simulink model "sldemo_suspn_3dof"  (R2018a)
settings: Solver=ode45  StartTime=0.0  StopTime=100  MaxStep=0.001  RelTol=1e-3  AbsTol=1e-6
PreLoadFcn:
  | sldemo_suspn_3dof_data
undefined symbols (not defined in the file or in its folder): Cr, g, Ixx, Iyy, Kf, Kr, L, Mb, sigbuilder_block, W
Description:
  | Automotive Suspension
  | 
  | This demo describes a simplified car suspension model in three degrees of
  | freedom (DoF): pitch, yaw and vertical displacement. The demo provides a description of the model to
  | show how simulation can be used for investigating ride characteristics. The Signal Builder block was used to
  | capture different road profiles to test the suspension against.
settings Model: FPTRunName=Active  ModifiedByFormat=The MathWorks Inc.  ExtModeTrigMode=oneshot  ExtModeArmWhenConnect=off  ExtModeAutoUpdateStatusClock=off  TunableVars=Cf,Mb  TunableVarsStorageClass=Auto,Auto  TunableVarsTypeQualifier=,  Creator=The MathWorks, Inc.  LastModifiedBy=The MathWorks Inc.
settings SolverCC: AutoScaleAbsTol=off
settings DataIOCC: InitialState=x0  SaveFormat=Array  SaveOutput=off  DSMLogging=off  SaveTime=off  ReturnWorkspaceOutputs=on  StateSaveName=x  ReturnWorkspaceOutputsName=simout
settings OptimizationCC: BooleanDataType=off  DefaultParameterBehavior=Inlined  InlineInvariantSignals=on  ExpressionDepthLimit=2147483647  InitFltsAndDblsToZero=on  LifeSpan=inf  BufferReusableBoundary=off
settings DebuggingCC: SaveWithParameterizedLinksMsg=none  SignalResolutionControl=TryResolveAllWithWarning  MultiTaskDSMMsg=warning  SigSpecEnsureSampleTimeMsg=none  IntegerOverflowMsg=none  FcnCallInpInsideContextMsg=warning  BusObjectLabelMismatch=none  StateNameClashWarn=warning  SFUnexpectedBacktrackingDiag=warning  SFNoUnconditionalDefaultTransitionDiag=warning  SFExecutionAtInitializationDiag=none  IntegerSaturationMsg=none
settings HardwareCC: ProdBitPerPointer=32  ProdBitPerSizeT=32  ProdBitPerPtrDiffT=32  ProdLargestAtomicFloat=None  ProdIntDivRoundTo=Undefined  ProdEndianess=Unspecified  ProdWordSize=32  ProdHWDeviceType=32-bit Generic
settings ModelReferenceCC: PropagateSignalLabelsOutOfModel=off
settings RTWCC: Description=Generic Real-Time Target
settings CodeAppCC: StateflowObjectComments=on
settings GRTTargetCC: TargetFcnLib=ansi_tfl_tmw.mat  TargetLangStandard=C89/C90 (ANSI)  GeneratePreprocessorConditionals=Disable all  CombineOutputUpdateFcns=off  GRTInterface=on
settings ConfigComp: CovMetricSettings=dw  CovHtmlReporting=on  CovSaveCumulativeToWorkspaceVar=on  CovSaveSingleToWorkspaceVar=on  CovExternalEMLEnable=off  CovSFcnEnable=off

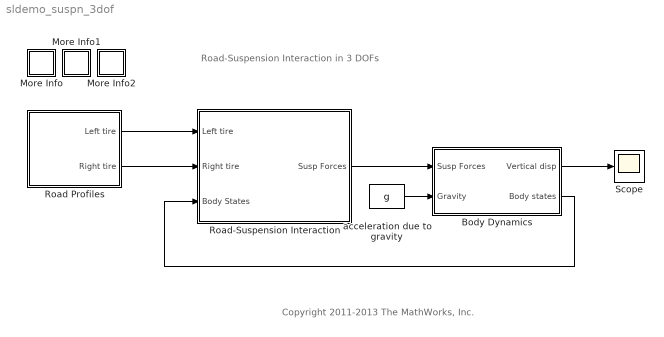
== system sldemo_suspn_3dof ==
  note: Road-Suspension Interaction in 3 DOFs
  note: Copyright 2011-2013 The MathWorks, Inc.
  Body Dynamics : Subsystem
  More Info : Subsystem
      settings: OpenFcn=helpview(fullfile(docroot,'simulink','helptargets.map'),'sldemo_parsim_testcase_suspn');
      mask Display: disp('?')
  More Info1 : Subsystem
      settings: OpenFcn=helpview(fullfile(docroot,'simulink','helptargets.map'),'sldemo_parsim_paramsweep_suspn');
      mask Display: disp('?')
  More Info2 : Subsystem
      settings: OpenFcn=helpview(fullfile(docroot,'simulink','helptargets.map'),'sldemo_parsim_paramsweep_suspn_raccel');
      mask Display: disp('?')
  Road Profiles : Subsystem  Tag=STV Subsys  LoadFcn=sigbuilder_block('load');  StartFcn=sigbuilder_block('start');  StopFcn=sigbuilder_block('stop');  ClipboardFcn=sigbuilder_block('clipboard');  mask(Sigbuilder block){tuvar=[0:10]}
      mask help: Create and generate interchangeable groups of signals whose waveforms are piecewise linear.
      mask init:
      | if ~strcmp(get_param(bdroot(gcbh),'SimulationStatus'),'stopped') tuvar = sigbuilder_block('maskInit'); end
      settings: CopyFcn=sigbuilder_block('copy');  DeleteFcn=sigbuilder_block('delete');  ModelCloseFcn=sigbuilder_block('modelClose');  PreSaveFcn=sigbuilder_block('preSave');  PauseFcn=sigbuilder_block('pause')  ContinueFcn=sigbuilder_block('continue')  NameChangeFcn=sigbuilder_block('namechange');  OpenFcn=sigbuilder_block('open',[108.621 149.586 549.931 399.724 ]);  CloseFcn=sigbuilder_block('close');
      mask Display: plot(0, 0, 100, 100,[2, 2, 32, 32, 2], [68, 8, 8, 68, 68],[32, 2], [38, 38], [32, 19, 2],[53, 60, 44], [32, 17, 17, 2],[16, 16, 31, 31]);txt = getActiveGroup(gcbh);text(2, 100, txt,'verticalAlignment', 'top');
  Road-Suspension Interaction : Subsystem  mask{Kf=Kf, Cf=150, Kr=Kr, Cr=Cr}
      mask prompts: Kf "Front susp. stiffness"; Cf "Front susp. damping"; Kr "Rear susp. stiffness"; Cr "Rear susp. damping"
  Scope : Scope
  acceleration due to gravity : Constant  Value=g
  wires:
  Road-Suspension Interaction/1(Susp Forces) -> Body Dynamics/1(Susp Forces)
  Road Profiles/1(Left tire) -> Road-Suspension Interaction/1("Left tire ")
  Road Profiles/2(Right tire) -> Road-Suspension Interaction/2(Right tire)
  Body Dynamics/2(Body states) -> Road-Suspension Interaction/3(Body States)
  Body Dynamics/1(Vertical disp) -> Scope/1
  acceleration due to gravity/1 -> Body Dynamics/2(Gravity)

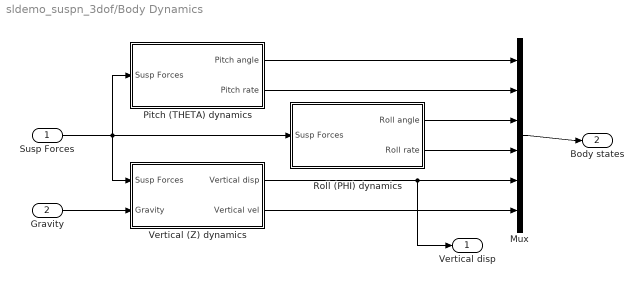
== system sldemo_suspn_3dof/Body Dynamics ==
  Susp Forces : Inport
  Gravity : Inport  Port=2
  Mux : Mux  Inputs=6
  Pitch (THETA) dynamics : Subsystem
  Roll (PHI) dynamics : Subsystem
  Vertical (Z) dynamics : Subsystem
  Vertical disp : Outport
  Body states : Outport  Port=2
  wires:
  Mux/1 -> Body states/1
  Pitch (THETA) dynamics/1(Pitch angle) -> Mux/1
  Pitch (THETA) dynamics/2(Pitch rate) -> Mux/2
  Roll (PHI) dynamics/1(Roll angle) -> Mux/3
  Roll (PHI) dynamics/2(Roll rate) -> Mux/4
  Vertical (Z) dynamics/1(Vertical disp) -> Mux/5, Vertical disp/1
  Vertical (Z) dynamics/2(Vertical vel) -> Mux/6
  Susp Forces/1 -> Pitch (THETA) dynamics/1(Susp Forces), Roll (PHI) dynamics/1(Susp Forces), Vertical (Z) dynamics/1(Susp Forces)
  Gravity/1 -> Vertical (Z) dynamics/2(Gravity)

== system sldemo_suspn_3dof/More Info ==

== system sldemo_suspn_3dof/More Info1 ==

== system sldemo_suspn_3dof/More Info2 ==

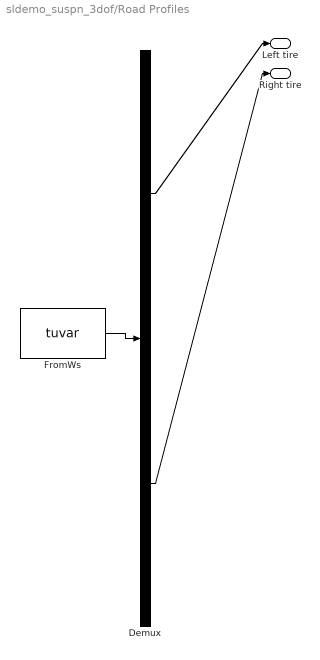
== system sldemo_suspn_3dof/Road Profiles ==
  Demux : Demux  Tag=STV Demux  Outputs=2
  FromWs : FromWorkspace  Tag=STV FromWs  VariableName=tuvar  SampleTime=0  OutputAfterFinalValue=Setting to zero
      SigBuilderData=|
      | common.afterFinalStr = 'Set to zero'
      | common.sampleTime = '0'
      | dataSet(1).timeRange = [0 102.3]
      | dataSet(1).name = 'Road1'
      | dataSet(2).timeRange = [0 102.3]
      | dataSet(2).name = 'Road2'
      | dataSet(3).timeRange = [0 102.3]
      | dataSet(3).name = 'Road3'
      | dataSet(4).timeRange = [0 102.3]
      | dataSet(4).name = 'Road4'
      | dataSet(5).timeRange = [0 102.3]
      | dataSet(5).name = 'Road5'
      | dataSet(6).timeRange = [0 102.3]
      | dataSet(6).name = 'Road6'
      | dataSet(7).timeRange = [0 102.3]
      | dataSet(7).name = 'Road7'
      | dataSet(8).timeRange = [0 102.3]
      | dataSet(8).name = 'Road8'
      | dataSet(9).timeRange = [0 102.3]
      | dataSet(9).name = 'Road9'
      | dataSet(10).timeRange = [0 102.3]
      | dataSet(10).name = 'Road10'
      | dataSet(11).timeRange = [0 102.3]
      | dataSet(11).name = 'Road11'
      | dataSet(12).timeRange = [0 102.3]
      | dataSet(12).name = 'Road12'
      | dataSet(13).timeRange = [0 102.3]
      | dataSet(13).name = 'Road13'
      | dataSet(14).timeRange = [0 102.3]
      | dataSet(14).name = 'Road14'
      | dataSet(15).timeRange = [0 102.3]
      | dataSet(15).name = 'Road15'
      | dataSet(16).timeRange = [0 102.3]
      | dataSet(16).name = 'Road16'
      | dataSet(17).timeRange = [0 102.3]
      | dataSet(17).name = 'Road17'
      | dataSet(18).timeRange = [0 102.3]
      | dataSet(18).name = 'Road18'
      | dataSet(19).timeRange = [0 102.3]
      | dataSet(19).name = 'Road19'
      | dataSet(20).timeRange = [0 102.3]
      | dataSet(20).name = 'Road20'
      | sbobj.Name = 'Signal Builder'
      | sbobj.Groups(1).Name = 'Road1'
      | sbobj.Groups(1).Signals(1).Name = 'Left tire'
      | sbobj.Groups(1).Signals(1).XData = [0 0.1 0.2 0.3 0.4 0.5 0.6 0.7 0.8 0.9 1 1.1 ... (1024 elements, 1x1024)]
      | sbobj.Groups(1).Signals(1).YData = [0.00473211644634 0.00467440555502 0.00464410099502 0.00454324182484 0.00445514799148 0.0043326490208 0.00423785066412 0.0042993177206 0.00422544735533 0.00410809626891 0.00412946729868 0.00411767616593 ... (1024 elements, 1x1024)]
      | sbobj.Groups(1).Signals(2).Name = 'Right tire'
      | sbobj.Groups(1).Signals(2).XData = [0 0.1 0.2 0.3 0.4 0.5 0.6 0.7 0.8 0.9 1 1.1 ... (1024 elements, 1x1024)]
      | sbobj.Groups(1).Signals(2).YData = [0.00528049577434 0.00509711727989 0.00506446595634 0.00501214877729 0.00490088724648 0.0049331354282 0.00486498626463 0.00475766732988 0.0047835078559 0.00468735204086 0.00453387383384 0.00439901634932 ... (1024 elements, 1x1024)]
      | sbobj.Groups(1).TimeRange = [0 102.3]
      | sbobj.Groups(2).Name = 'Road2'
      | sbobj.Groups(2).Signals(1).Name = 'Left tire'
      | sbobj.Groups(2).Signals(1).XData = [0 0.1 0.2 0.3 0.4 0.5 0.6 0.7 0.8 0.9 1 1.1 ... (1024 elements, 1x1024)]
      | sbobj.Groups(2).Signals(1).YData = [-0.00302076151696 -0.00288652811099 -0.00307685510952 -0.00307502876534 -0.00324446782403 -0.00331553430871 -0.00334240017969 -0.00326247309041 -0.00316856911182 -0.00296957686299 -0.0027554885003 -0.00258448600687 ... (1024 elements, 1x1024)]
      | sbobj.Groups(2).Signals(2).Name = 'Right tire'
      | sbobj.Groups(2).Signals(2).XData = [0 0.1 0.2 0.3 0.4 0.5 0.6 0.7 0.8 0.9 1 1.1 ... (1024 elements, 1x1024)]
      | sbobj.Groups(2).Signals(2).YData = [-0.00201835921981 -0.00193048581992 -0.00176056859737 -0.0016439537928 -0.00144888110683 -0.00159615113793 -0.00171506406145 -0.00153884382486 -0.00141895285376 -0.00142872348877 -0.00145512582738 -0.00139669902584 ... (1024 elements, 1x1024)]
      | sbobj.Groups(2).TimeRange = [0 102.3]
      | sbobj.Groups(3).Name = 'Road3'
      | sbobj.Groups(3).Signals(1).Name = 'Left tire'
      | sbobj.Groups(3).Signals(1).XData = [0 0.1 0.2 0.3 0.4 0.5 0.6 0.7 0.8 0.9 1 1.1 ... (1024 elements, 1x1024)]
      | sbobj.Groups(3).Signals(1).YData = [0.00292193601345 0.00277798330516 0.00264852811019 0.00269353298318 0.00260613635012 0.00268824973072 0.00268899858507 0.00266903047874 0.00251936938684 0.00231497901336 0.00237012995803 0.00231547478993 ... (1024 elements, 1x1024)]
      | sbobj.Groups(3).Signals(2).Name = 'Right tire'
      | sbobj.Groups(3).Signals(2).XData = [0 0.1 0.2 0.3 0.4 0.5 0.6 0.7 0.8 0.9 1 1.1 ... (1024 elements, 1x1024)]
      | sbobj.Groups(3).Signals(2).YData = [0.00268504042027 0.00266079424453 0.00249731950168 0.00247212354596 0.00237415879272 0.00219229196121 0.00204171306183 0.00198473585189 0.00188648751614 0.00193081127734 0.0017234922974 0.00154980466048 ... (1024 elements, 1x1024)]
      | sbobj.Groups(3).TimeRange = [0 102.3]
      | sbobj.Groups(4).Name = 'Road4'
      | sbobj.Groups(4).Signals(1).Name = 'Left tire'
      | sbobj.Groups(4).Signals(1).XData = [0 0.1 0.2 0.3 0.4 0.5 0.6 0.7 0.8 0.9 1 1.1 ... (1024 elements, 1x1024)]
      | sbobj.Groups(4).Signals(1).YData = [0.00616079209813 0.00638852668327 0.0067000308695 0.00700469605804 0.00722755687693 0.00740916655576 0.00732138086583 0.00752365486656 0.00767138035593 0.007682048414 0.00782576749353 0.00797441933197 ... (1024 elements, 1x1024)]
      | sbobj.Groups(4).Signals(2).Name = 'Right tire'
      | sbobj.Groups(4).Signals(2).XData = [0 0.1 0.2 0.3 0.4 0.5 0.6 0.7 0.8 0.9 1 1.1 ... (1024 elements, 1x1024)]
      | sbobj.Groups(4).Signals(2).YData = [0.00745096656951 0.00748223108095 0.00743938160251 0.00756617671073 0.00772313585198 0.00805109398319 0.00829111604762 0.00855264761538 0.00871988520703 0.00872848787177 0.00862440573102 0.00888785524686 ... (1024 elements, 1x1024)]
      | sbobj.Groups(4).TimeRange = [0 102.3]
      | sbobj.Groups(5).Name = 'Road5'
      | sbobj.Groups(5).Signals(1).Name = 'Left tire'
      | sbobj.Groups(5).Signals(1).XData = [0 0.1 0.2 0.3 0.4 0.5 0.6 0.7 0.8 0.9 1 1.1 ... (1024 elements, 1x1024)]
      | sbobj.Groups(5).Signals(1).YData = [0.000554066239591 0.000793708867367 0.000871588264979 0.0010608183551 0.00127043504725 0.00126617829925 0.00113472652318 0.00111735061431 0.00108568677788 0.000954073484207 0.000725297690323 0.000569951055391 ... (1024 elements, 1x1024)]
      | sbobj.Groups(5).Signals(2).Name = 'Right tire'
      | sbobj.Groups(5).Signals(2).XData = [0 0.1 0.2 0.3 0.4 0.5 0.6 0.7 0.8 0.9 1 1.1 ... (1024 elements, 1x1024)]
      | sbobj.Groups(5).Signals(2).YData = [0.00135212139139 0.00117515083497 0.00102384774237 0.00101503793836 0.000937905766135 0.000936234035331 0.000942025020523 0.000944636497011 0.000930027392227 0.000749819221585 0.000727989024936 0.000621825438773 ... (1024 elements, 1x1024)]
      | sbobj.Groups(5).TimeRange = [0 102.3]
      | sbobj.Groups(6).Name = 'Road6'
      | sbobj.Groups(6).Signals(1).Name = 'Left tire'
      | sbobj.Groups(6).Signals(1).XData = [0 0.1 0.2 0.3 0.4 0.5 0.6 0.7 0.8 0.9 1 1.1 ... (1024 elements, 1x1024)]
      | sbobj.Groups(6).Signals(1).YData = [0.00153774999396 0.00154455487736 0.000925956904154 0.000243851099195 0.000797909036254 0.00022254178888 0.000293931713738 0.0013287345336 0.00104349828299 0.000951361881332 0.000595257082134 0.000816695497374 ... (1024 elements, 1x1024)]
      | sbobj.Groups(6).Signals(2).Name = 'Right tire'
      | sbobj.Groups(6).Signals(2).XData = [0 0.1 0.2 0.3 0.4 0.5 0.6 0.7 0.8 0.9 1 1.1 ... (1024 elements, 1x1024)]
      | sbobj.Groups(6).Signals(2).YData = [0.000494774793197 0.000549431793974 0.000426624713092 0.000686597782016 0.000473613268552 0.000643650437596 5.56323455251e-05 0.000239173096508 -6.19023823402e-05 -0.000596655061178 -0.000827633762604 -0.000337467053855 ... (1024 elements, 1x1024)]
      | sbobj.Groups(6).TimeRange = [0 102.3]
      | sbobj.Groups(7).Name = 'Road7'
      | sbobj.Groups(7).Signals(1).Name = 'Left tire'
      | sbobj.Groups(7).Signals(1).XData = [0 0.1 0.2 0.3 0.4 0.5 0.6 0.7 0.8 0.9 1 1.1 ... (1024 elements, 1x1024)]
      | sbobj.Groups(7).Signals(1).YData = [0.00466211800598 0.00467773753959 0.00462172232334 0.00555135602106 0.00513121634954 0.00613380739552 0.00556485337031 0.00573789876241 0.00605930510884 0.00539494795418 0.00607671461587 0.00548943337417 ... (1024 elements, 1x1024)]
      | sbobj.Groups(7).Signals(2).Name = 'Right tire'
      | sbobj.Groups(7).Signals(2).XData = [0 0.1 0.2 0.3 0.4 0.5 0.6 0.7 0.8 0.9 1 1.1 ... (1024 elements, 1x1024)]
      | sbobj.Groups(7).Signals(2).YData = [0.0042013095511 0.00485695391815 0.0041131940406 0.00375090747664 0.00386429706123 0.00475688806169 0.00496870049203 0.00491391514981 0.00559214957707 0.00571237046815 0.0045301820995 0.00509399466091 ... (1024 elements, 1x1024)]
      | sbobj.Groups(7).TimeRange = [0 102.3]
      | sbobj.Groups(8).Name = 'Road8'
      | sbobj.Groups(8).Signals(1).Name = 'Left tire'
      | sbobj.Groups(8).Signals(1).XData = [0 0.1 0.2 0.3 0.4 0.5 0.6 0.7 0.8 0.9 1 1.1 ... (1024 elements, 1x1024)]
      | sbobj.Groups(8).Signals(1).YData = [0.00758913226527 0.00754692345972 0.00752658169702 0.00765873482654 0.00725381421444 0.00744810927045 0.00773690222317 0.00762087397962 0.00781872158319 0.00738448703918 0.0075931621737 0.00752147382619 ... (1024 elements, 1x1024)]
      | sbobj.Groups(8).Signals(2).Name = 'Right tire'
      | sbobj.Groups(8).Signals(2).XData = [0 0.1 0.2 0.3 0.4 0.5 0.6 0.7 0.8 0.9 1 1.1 ... (1024 elements, 1x1024)]
      | sbobj.Groups(8).Signals(2).YData = [0.00838905488672 0.00875461793738 0.00901655269553 0.00839254635776 0.00790744440481 0.00805603356054 0.00832594345385 0.00850280913193 0.00806336473748 0.00819057465251 0.00726246977162 0.00759134311203 ... (1024 elements, 1x1024)]
      | sbobj.Groups(8).TimeRange = [0 102.3]
      | sbobj.Groups(9).Name = 'Road9'
      | sbobj.Groups(9).Signals(1).Name = 'Left tire'
      | sbobj.Groups(9).Signals(1).XData = [0 0.1 0.2 0.3 0.4 0.5 0.6 0.7 0.8 0.9 1 1.1 ... (1024 elements, 1x1024)]
      | sbobj.Groups(9).Signals(1).YData = [0.00545944368639 0.00582668704816 0.00617047160024 0.00557147660936 0.00575804646647 0.0055149206281 0.00572610782593 0.0059053666758 0.00548260210233 0.00561969157093 0.0054496756372 0.0061077350342 ... (1024 elements, 1x1024)]
      | sbobj.Groups(9).Signals(2).Name = 'Right tire'
      | sbobj.Groups(9).Signals(2).XData = [0 0.1 0.2 0.3 0.4 0.5 0.6 0.7 0.8 0.9 1 1.1 ... (1024 elements, 1x1024)]
      | sbobj.Groups(9).Signals(2).YData = [0.0041341680497 0.00424806598971 0.00405728028022 0.00450572841426 0.00363231320765 0.00376496647699 0.00449256861668 0.0049144731951 0.00482833729881 0.00484842910869 0.00579906791572 0.00501282723811 ... (1024 elements, 1x1024)]
      | sbobj.Groups(9).TimeRange = [0 102.3]
      | sbobj.Groups(10).Name = 'Road10'
      | sbobj.Groups(10).Signals(1).Name = 'Left tire'
      | sbobj.Groups(10).Signals(1).XData = [0 0.1 0.2 0.3 0.4 0.5 0.6 0.7 0.8 0.9 1 1.1 ... (1024 elements, 1x1024)]
      | sbobj.Groups(10).Signals(1).YData = [-0.0144751087058 -0.0138480187327 -0.0135089408218 -0.0133963442669 -0.0135987059564 -0.0132544277135 -0.0139868746694 -0.0134572838224 -0.0131045012422 -0.0130857589569 -0.0121116376232 -0.0121703441668 ... (1024 elements, 1x1024)]
      | sbobj.Groups(10).Signals(2).Name = 'Right tire'
      | sbobj.Groups(10).Signals(2).XData = [0 0.1 0.2 0.3 0.4 0.5 0.6 0.7 0.8 0.9 1 1.1 ... (1024 elements, 1x1024)]
      | sbobj.Groups(10).Signals(2).YData = [-0.0132991630261 -0.0137672255646 -0.0134012844979 -0.0135978101072 -0.0134329129204 -0.0123268000989 -0.0118650041533 -0.0119084971541 -0.0126712272709 -0.0116830867475 -0.0109118533732 -0.0112171924526 ... (1024 elements, 1x1024)]
      | sbobj.Groups(10).TimeRange = [0 102.3]
      | sbobj.Groups(11).Name = 'Road11'
      | sbobj.Groups(11).Signals(1).Name = 'Left tire'
      | sbobj.Groups(11).Signals(1).XData = [0 0.1 0.2 0.3 0.4 0.5 0.6 0.7 0.8 0.9 1 1.1 ... (1024 elements, 1x1024)]
      | sbobj.Groups(11).Signals(1).YData = [0.000136881298967 0.000357736458052 0.000393728673989 0.000441850869331 0.000463330868559 0.000436864644761 0.000546301647008 0.000633409993691 0.000779640551224 0.000917640996056 0.000957457218823 0.00112343221137 ... (1024 elements, 1x1024)]
      | sbobj.Groups(11).Signals(2).Name = 'Right tire'
      | sbobj.Groups(11).Signals(2).XData = [0 0.1 0.2 0.3 0.4 0.5 0.6 0.7 0.8 0.9 1 1.1 ... (1024 elements, 1x1024)]
      | sbobj.Groups(11).Signals(2).YData = [0.000273088846773 0.000278825033991 0.000396833475121 0.000483461336575 0.00056215306635 0.000715169629702 0.000866422630103 0.00103940104465 0.00113438156799 0.00131464938322 0.00137789478615 0.00151561832404 ... (1024 elements, 1x1024)]
      | sbobj.Groups(11).TimeRange = [0 102.3]
      | sbobj.Groups(12).Name = 'Road12'
      | sbobj.Groups(12).Signals(1).Name = 'Left tire'
      | sbobj.Groups(12).Signals(1).XData = [0 0.1 0.2 0.3 0.4 0.5 0.6 0.7 0.8 0.9 1 1.1 ... (1024 elements, 1x1024)]
      | sbobj.Groups(12).Signals(1).YData = [0.00789178064295 0.00781260152005 0.00781810111865 0.00796365444698 0.00784712616122 0.00786211429938 0.00791307970479 0.00792233212523 0.00798013684222 0.00812266609699 0.00827118867259 0.0082727880223 ... (1024 elements, 1x1024)]
      | sbobj.Groups(12).Signals(2).Name = 'Right tire'
      | sbobj.Groups(12).Signals(2).XData = [0 0.1 0.2 0.3 0.4 0.5 0.6 0.7 0.8 0.9 1 1.1 ... (1024 elements, 1x1024)]
      | sbobj.Groups(12).Signals(2).YData = [0.00685163464958 0.00683055981156 0.00693131975999 0.00704129721591 0.00703599483142 0.00708318375949 0.00724761124181 0.00726613432561 0.00728219713307 0.00738604304843 0.00738709934486 0.00750010822148 ... (1024 elements, 1x1024)]
      | sbobj.Groups(12).TimeRange = [0 102.3]
      | sbobj.Groups(13).Name = 'Road13'
      | sbobj.Groups(13).Signals(1).Name = 'Left tire'
      | sbobj.Groups(13).Signals(1).XData = [0 0.1 0.2 0.3 0.4 0.5 0.6 0.7 0.8 0.9 1 1.1 ... (1024 elements, 1x1024)]
      | sbobj.Groups(13).Signals(1).YData = [-0.0121388620143 -0.0120426805628 -0.0120718282771 -0.012033200691 -0.0117728297154 -0.0115002638537 -0.0113794230031 -0.0112698021669 -0.0111471171106 -0.0110907264407 -0.0109970335901 -0.0110427719501 ... (1024 elements, 1x1024)]
      | sbobj.Groups(13).Signals(2).Name = 'Right tire'
      | sbobj.Groups(13).Signals(2).XData = [0 0.1 0.2 0.3 0.4 0.5 0.6 0.7 0.8 0.9 1 1.1 ... (1024 elements, 1x1024)]
      | sbobj.Groups(13).Signals(2).YData = [-0.0114798456104 -0.0113933856875 -0.0113436421112 -0.0111249408988 -0.011128298253 -0.0109139409458 -0.010793276881 -0.010696041257 -0.0106004556665 -0.0105166007438 -0.0105545515975 -0.0105411628631 ... (1024 elements, 1x1024)]
      | sbobj.Groups(13).TimeRange = [0 102.3]
      | sbobj.Groups(14).Name = 'Road14'
      | sbobj.Groups(14).Signals(1).Name = 'Left tire'
      | sbobj.Groups(14).Signals(1).XData = [0 0.1 0.2 0.3 0.4 0.5 0.6 0.7 0.8 0.9 1 1.1 ... (1024 elements, 1x1024)]
      | sbobj.Groups(14).Signals(1).YData = [0.0180895391114 0.0181839420272 0.0183373780546 0.0184185273621 0.0185926784748 0.0187008411222 0.0189828278539 0.0191973159812 0.0195193678526 0.0196414264908 0.0197683277438 0.0198991759403 ... (1024 elements, 1x1024)]
      | sbobj.Groups(14).Signals(2).Name = 'Right tire'
      | sbobj.Groups(14).Signals(2).XData = [0 0.1 0.2 0.3 0.4 0.5 0.6 0.7 0.8 0.9 1 1.1 ... (1024 elements, 1x1024)]
      | sbobj.Groups(14).Signals(2).YData = [0.0181852267494 0.0182686615537 0.0183516262967 0.0185187800225 0.0185825348553 0.0186448979921 0.0186433257675 0.0187515231655 0.0187646382675 0.0189736634747 0.0190565884772 0.0191951790755 ... (1024 elements, 1x1024)]
      | sbobj.Groups(14).TimeRange = [0 102.3]
      | sbobj.Groups(15).Name = 'Road15'
      | sbobj.Groups(15).Signals(1).Name = 'Left tire'
      | sbobj.Groups(15).Signals(1).XData = [0 0.1 0.2 0.3 0.4 0.5 0.6 0.7 0.8 0.9 1 1.1 ... (1024 elements, 1x1024)]
      | sbobj.Groups(15).Signals(1).YData = [-0.0106511001183 -0.0107656990312 -0.0107737952176 -0.0107094335786 -0.0107471431332 -0.010604994661 -0.0104942842738 -0.0105249711755 -0.0104209141567 -0.0103747514325 -0.010276252305 -0.0102354900668 ... (1024 elements, 1x1024)]
      | sbobj.Groups(15).Signals(2).Name = 'Right tire'
      | sbobj.Groups(15).Signals(2).XData = [0 0.1 0.2 0.3 0.4 0.5 0.6 0.7 0.8 0.9 1 1.1 ... (1024 elements, 1x1024)]
      | sbobj.Groups(15).Signals(2).YData = [-0.0095307867657 -0.00956880544118 -0.00959530412329 -0.00962274183777 -0.00978413229659 -0.00971053624683 -0.00961639091988 -0.00957113170828 -0.00970459834661 -0.00983845749568 -0.00997276037227 -0.0100131637618 ... (1024 elements, 1x1024)]
      | sbobj.Groups(15).TimeRange = [0 102.3]
      | sbobj.Groups(16).Name = 'Road16'
      | sbobj.Groups(16).Signals(1).Name = 'Left tire'
      | sbobj.Groups(16).Signals(1).XData = [0 0.1 0.2 0.3 0.4 0.5 0.6 0.7 0.8 0.9 1 1.1 ... (1024 elements, 1x1024)]
      | sbobj.Groups(16).Signals(1).YData = [0.0463931826849 0.0473311861089 0.0467107761858 0.0455277975911 0.0451084544958 0.045895154642 0.0441598783404 0.0431662667549 0.0424286170792 0.0428720292654 0.043072925124 0.0429881759739 ... (1024 elements, 1x1024)]
      | sbobj.Groups(16).Signals(2).Name = 'Right tire'
      | sbobj.Groups(16).Signals(2).XData = [0 0.1 0.2 0.3 0.4 0.5 0.6 0.7 0.8 0.9 1 1.1 ... (1024 elements, 1x1024)]
      | sbobj.Groups(16).Signals(2).YData = [0.029754217561 0.0310911506439 0.0309881994972 0.0320808425478 0.0331260851946 0.0344002551069 0.0327461013478 0.0339867920912 0.0351549320475 0.0379268368575 0.038627204707 0.0409816951094 ... (1024 elements, 1x1024)]
      | sbobj.Groups(16).TimeRange = [0 102.3]
      | sbobj.Groups(17).Name = 'Road17'
      | sbobj.Groups(17).Signals(1).Name = 'Left tire'
      | sbobj.Groups(17).Signals(1).XData = [0 0.1 0.2 0.3 0.4 0.5 0.6 0.7 0.8 0.9 1 1.1 ... (1024 elements, 1x1024)]
      | sbobj.Groups(17).Signals(1).YData = [-0.0659460961507 -0.0657737017805 -0.0680780972317 -0.0662266692622 -0.0670915798418 -0.0663510273968 -0.0664410929528 -0.0672183580234 -0.0681572876756 -0.0679728162926 -0.0663904249741 -0.0673330808489 ... (1024 elements, 1x1024)]
      | sbobj.Groups(17).Signals(2).Name = 'Right tire'
      | sbobj.Groups(17).Signals(2).XData = [0 0.1 0.2 0.3 0.4 0.5 0.6 0.7 0.8 0.9 1 1.1 ... (1024 elements, 1x1024)]
      | sbobj.Groups(17).Signals(2).YData = [-0.0723654152433 -0.0719414030343 -0.0713075513069 -0.0709032462893 -0.0716110973724 -0.072375605033 -0.0732728968111 -0.0738732031217 -0.0733634692873 -0.0721983703892 -0.0710267255598 -0.0699869220664 ... (1024 elements, 1x1024)]
      | sbobj.Groups(17).TimeRange = [0 102.3]
      | sbobj.Groups(18).Name = 'Road18'
      | sbobj.Groups(18).Signals(1).Name = 'Left tire'
      | sbobj.Groups(18).Signals(1).XData = [0 0.1 0.2 0.3 0.4 0.5 0.6 0.7 0.8 0.9 1 1.1 ... (1024 elements, 1x1024)]
      | sbobj.Groups(18).Signals(1).YData = [-0.0416743114161 -0.0429521319269 -0.0414076251964 -0.0430156173481 -0.0442586945698 -0.0437103391887 -0.0433877570159 -0.0431284402102 -0.0438796744885 -0.0441275806765 -0.043525122919 -0.0438830252161 ... (1024 elements, 1x1024)]
      | sbobj.Groups(18).Signals(2).Name = 'Right tire'
      | sbobj.Groups(18).Signals(2).XData = [0 0.1 0.2 0.3 0.4 0.5 0.6 0.7 0.8 0.9 1 1.1 ... (1024 elements, 1x1024)]
      | sbobj.Groups(18).Signals(2).YData = [-0.0304256443325 -0.031145710653 -0.0313159814187 -0.0315233138853 -0.0332768542163 -0.0339904231285 -0.0345005605545 -0.0369658696176 -0.0368223884158 -0.0361987922382 -0.0385613374578 -0.0393117260498 ... (1024 elements, 1x1024)]
      | sbobj.Groups(18).TimeRange = [0 102.3]
      | sbobj.Groups(19).Name = 'Road19'
      | sbobj.Groups(19).Signals(1).Name = 'Left tire'
      | sbobj.Groups(19).Signals(1).XData = [0 0.1 0.2 0.3 0.4 0.5 0.6 0.7 0.8 0.9 1 1.1 ... (1024 elements, 1x1024)]
      | sbobj.Groups(19).Signals(1).YData = [-0.0319680129063 -0.0297334201085 -0.0310842565466 -0.0290732267024 -0.0277918222251 -0.028045015933 -0.0274159711883 -0.0271689004524 -0.0254152572191 -0.0241541099631 -0.0262566563185 -0.0254770871175 ... (1024 elements, 1x1024)]
      | sbobj.Groups(19).Signals(2).Name = 'Right tire'
      | sbobj.Groups(19).Signals(2).XData = [0 0.1 0.2 0.3 0.4 0.5 0.6 0.7 0.8 0.9 1 1.1 ... (1024 elements, 1x1024)]
      | sbobj.Groups(19).Signals(2).YData = [-0.0214828498394 -0.0191391006723 -0.019055049233 -0.0209359350395 -0.0209075330992 -0.0201904789647 -0.0204015571228 -0.0184057758458 -0.0191205150769 -0.0173035901216 -0.0179448663042 -0.0156149760397 ... (1024 elements, 1x1024)]
      | sbobj.Groups(19).TimeRange = [0 102.3]
      | sbobj.Groups(20).Name = 'Road20'
      | sbobj.Groups(20).Signals(1).Name = 'Left tire'
      | sbobj.Groups(20).Signals(1).XData = [0 0.1 0.2 0.3 0.4 0.5 0.6 0.7 0.8 0.9 1 1.1 ... (1024 elements, 1x1024)]
      | sbobj.Groups(20).Signals(1).YData = [0.0562062983641 0.0573030401656 0.0570087628686 0.0566847164003 0.0575296235315 0.0564136527339 0.0561220637562 0.0581332751723 0.058172108212 0.0573686779096 0.0557002159126 0.0564551973097 ... (1024 elements, 1x1024)]
      | sbobj.Groups(20).Signals(2).Name = 'Right tire'
      | sbobj.Groups(20).Signals(2).XData = [0 0.1 0.2 0.3 0.4 0.5 0.6 0.7 0.8 0.9 1 1.1 ... (1024 elements, 1x1024)]
      | sbobj.Groups(20).Signals(2).YData = [0.0415752184371 0.0405808838241 0.0420636597295 0.0397581403296 0.0392167944078 0.0395929366966 0.0403277764692 0.0379173313525 0.0370146939845 0.037608344306 0.0380897634361 0.0379385762952 ... (1024 elements, 1x1024)]
      | sbobj.Groups(20).TimeRange = [0 102.3]
  Left tire : Outport  Tag=STV Outport
  Right tire : Outport  Tag=STV Outport  Port=2
  wires:
  Demux/1 -> Left tire/1
  FromWs/1 -> Demux/1
  Demux/2 -> Right tire/1

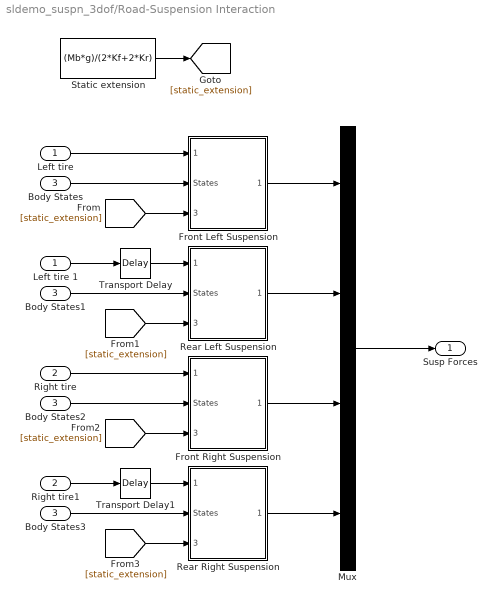
== system sldemo_suspn_3dof/Road-Suspension Interaction ==
  "Left tire " : Inport
  Right tire : Inport  Port=2
  Body States : Inport  Port=3
  Body States1 : InportShadow  Port=3
  Body States2 : InportShadow  Port=3
  Body States3 : InportShadow  Port=3
  Front Left Suspension : Subsystem  mask(half-car suspension){K=Kf, C=Cf}
      mask prompts: K "Stiffness = spring rate:"; C "Damping rate:"
      mask help:
      | Half-Car Suspension
      | The spring and damping rates for an individual wheel are entered below.  Their combined effect as applied to two wheels at the specified distance from the center of mass is computed.  The distance should be specified as positive if the subsystem is oriented such that increasing z corresponds to increasing theta, negative otherwise.
      mask Help: See "Using Simulink and Stateflow in Automotive Applications" for a mathematical derivation of the subsystem operation.  Contact your MathWorks distributor to obtain a copy.
      mask Display: plot(-1, 0, 13, 12, [1 12], [11 11], [1 5], [2 2], [1 2], [4.5 5], [2 0], [5 6], [0 2], [6 7], [2 0], [7 8], [0 1], [8 8.5], [1 1], [8.5 11], [1 1], [2 4.5], [5 5], [2 5], [4 6], [5 5], [4 4], [5 8], [6 6], [5 8], [4 6], [6.5 6.5], [5 5], [6.5 11], [0 1], [1 2], [2 3], [1 2], [4 5], [1 2])
  Front Right Suspension : Subsystem  mask(half-car suspension){K=Kf, C=Cf}
      mask prompts: K "Stiffness = spring rate:"; C "Damping rate:"
      mask help:
      | Half-Car Suspension
      | The spring and damping rates for an individual wheel are entered below.  Their combined effect as applied to two wheels at the specified distance from the center of mass is computed.  The distance should be specified as positive if the subsystem is oriented such that increasing z corresponds to increasing theta, negative otherwise.
      mask Help: See "Using Simulink and Stateflow in Automotive Applications" for a mathematical derivation of the subsystem operation.  Contact your MathWorks distributor to obtain a copy.
      mask Display: plot(-1, 0, 13, 12, [1 12], [11 11], [1 5], [2 2], [1 2], [4.5 5], [2 0], [5 6], [0 2], [6 7], [2 0], [7 8], [0 1], [8 8.5], [1 1], [8.5 11], [1 1], [2 4.5], [5 5], [2 5], [4 6], [5 5], [4 4], [5 8], [6 6], [5 8], [4 6], [6.5 6.5], [5 5], [6.5 11], [0 1], [1 2], [2 3], [1 2], [4 5], [1 2])
  Left tire 1 : InportShadow
  Mux : Mux
  Rear Left Suspension : Subsystem  mask(half-car suspension){K=Kr, C=Cr}
      mask prompts: K "Stiffness = spring rate:"; C "Damping rate:"
      mask help:
      | Half-Car Suspension
      | The spring and damping rates for an individual wheel are entered below.  Their combined effect as applied to two wheels at the specified distance from the center of mass is computed.  The distance should be specified as positive if the subsystem is oriented such that increasing z corresponds to increasing theta, negative otherwise.
      mask Help: See "Using Simulink and Stateflow in Automotive Applications" for a mathematical derivation of the subsystem operation.  Contact your MathWorks distributor to obtain a copy.
      mask Display: plot(-1, 0, 13, 12, [1 12], [11 11], [1 5], [2 2], [1 2], [4.5 5], [2 0], [5 6], [0 2], [6 7], [2 0], [7 8], [0 1], [8 8.5], [1 1], [8.5 11], [1 1], [2 4.5], [5 5], [2 5], [4 6], [5 5], [4 4], [5 8], [6 6], [5 8], [4 6], [6.5 6.5], [5 5], [6.5 11], [0 1], [1 2], [2 3], [1 2], [4 5], [1 2])
  Rear Right Suspension : Subsystem  mask(half-car suspension){K=Kr, C=Cr}
      mask prompts: K "Stiffness = spring rate:"; C "Damping rate:"
      mask help:
      | Half-Car Suspension
      | The spring and damping rates for an individual wheel are entered below.  Their combined effect as applied to two wheels at the specified distance from the center of mass is computed.  The distance should be specified as positive if the subsystem is oriented such that increasing z corresponds to increasing theta, negative otherwise.
      mask Help: See "Using Simulink and Stateflow in Automotive Applications" for a mathematical derivation of the subsystem operation.  Contact your MathWorks distributor to obtain a copy.
      mask Display: plot(-1, 0, 13, 12, [1 12], [11 11], [1 5], [2 2], [1 2], [4.5 5], [2 0], [5 6], [0 2], [6 7], [2 0], [7 8], [0 1], [8 8.5], [1 1], [8.5 11], [1 1], [2 4.5], [5 5], [2 5], [4 6], [5 5], [4 4], [5 8], [6 6], [5 8], [4 6], [6.5 6.5], [5 5], [6.5 11], [0 1], [1 2], [2 3], [1 2], [4 5], [1 2])
  Right tire1 : InportShadow  Port=2
  Static extension : Constant  Value=(Mb*g)/(2*Kf+2*Kr)
  Transport Delay : TransportDelay  DelayTime=0.1
  Transport Delay1 : TransportDelay  DelayTime=0.1
  Susp Forces : Outport
  wires:
  Front Left Suspension/1(Vertical Force) -> Mux/1
  Front Right Suspension/1(Vertical Force) -> Mux/3
  Rear Left Suspension/1(Vertical Force) -> Mux/2
  Rear Right Suspension/1(Vertical Force) -> Mux/4
  "Left tire "/1 -> Front Left Suspension/1(Road Input)
  Mux/1 -> Susp Forces/1
  Left tire 1/1 -> Transport Delay/1
  Right tire1/1 -> Transport Delay1/1
  Body States/1 -> Front Left Suspension/2(States)
  Body States2/1 -> Front Right Suspension/2(States)
  Body States1/1 -> Rear Left Suspension/2(States)
  Transport Delay/1 -> Rear Left Suspension/1(Road Input)
  Right tire/1 -> Front Right Suspension/1(Road Input)
  Transport Delay1/1 -> Rear Right Suspension/1(Road Input)
  Body States3/1 -> Rear Right Suspension/2(States)
  Static extension/1 -> [static_extension]
  [static_extension] -> Front Left Suspension/3(Static ext.)
  [static_extension] -> Front Right Suspension/3(Static ext.)
  [static_extension] -> Rear Right Suspension/3(Static Ext.)
  [static_extension] -> Rear Left Suspension/3(Static Ext.)

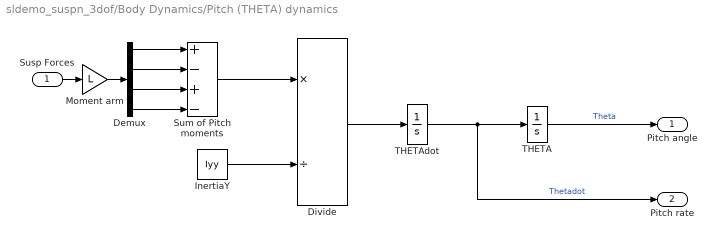
== system sldemo_suspn_3dof/Body Dynamics/Pitch (THETA) dynamics ==
  Susp Forces : Inport
  Demux : Demux
  Divide : Product  Inputs=*/
  InertiaY : Constant  Value=Iyy
  Moment arm : Gain  Gain=L
  Sum of Pitch moments : Sum  Inputs=+-+-
  THETA : Integrator  InitialCondition=-8.7e-20
  THETAdot : Integrator  InitialCondition=8.04e-28
  Pitch angle : Outport
  Pitch rate : Outport  Port=2
  wires:
  Divide/1 -> THETAdot/1
  THETAdot/1 -> THETA/1, Pitch rate/1  "Thetadot"
  Sum of Pitch moments/1 -> Divide/1
  THETA/1 -> Pitch angle/1  "Theta"
  Susp Forces/1 -> Moment arm/1
  Moment arm/1 -> Demux/1
  Demux/1 -> Sum of Pitch moments/1
  Demux/2 -> Sum of Pitch moments/2
  Demux/3 -> Sum of Pitch moments/3
  Demux/4 -> Sum of Pitch moments/4
  InertiaY/1 -> Divide/2

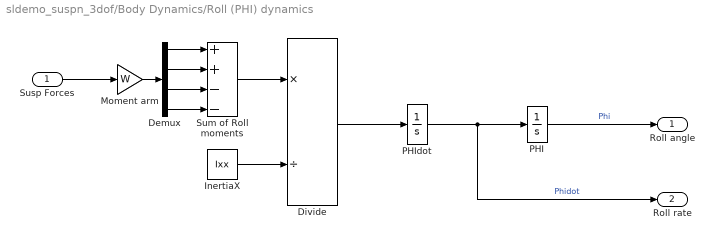
== system sldemo_suspn_3dof/Body Dynamics/Roll (PHI) dynamics ==
  Susp Forces : Inport
  Demux : Demux
  Divide : Product  Inputs=*/
  InertiaX : Constant  Value=Ixx
  Moment arm : Gain  Gain=W
  PHI : Integrator  InitialCondition=-8.7e-20
  PHIdot : Integrator  InitialCondition=8.04e-28
  Sum of Roll moments : Sum  Inputs=++--
  Roll angle : Outport
  Roll rate : Outport  Port=2
  wires:
  PHI/1 -> Roll angle/1  "Phi"
  PHIdot/1 -> Roll rate/1, PHI/1  "Phidot"
  Divide/1 -> PHIdot/1
  Moment arm/1 -> Demux/1
  Susp Forces/1 -> Moment arm/1
  Demux/1 -> Sum of Roll moments/1
  Demux/2 -> Sum of Roll moments/2
  Demux/3 -> Sum of Roll moments/3
  Demux/4 -> Sum of Roll moments/4
  Sum of Roll moments/1 -> Divide/1
  InertiaX/1 -> Divide/2

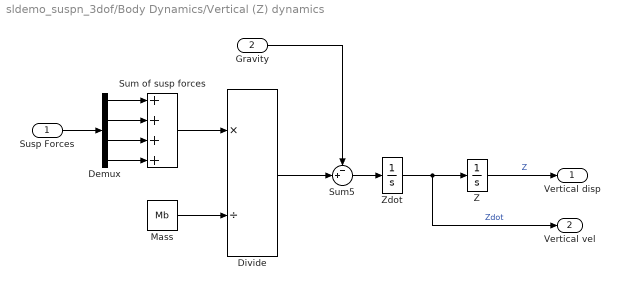
== system sldemo_suspn_3dof/Body Dynamics/Vertical (Z) dynamics ==
  Susp Forces : Inport
  Gravity : Inport  Port=2
  Demux : Demux
  Divide : Product  Inputs=*/
  Mass : Constant  Value=Mb
  Sum of susp forces : Sum  Inputs=++++
  Sum5 : Sum  Inputs=-+|  SaturateOnIntegerOverflow=on  InputSameDT=on  OutDataTypeStr=Inherit: Same as first input
  Z : Integrator
  Zdot : Integrator
  Vertical disp : Outport
  Vertical vel : Outport  Port=2
  wires:
  Sum5/1 -> Zdot/1
  Zdot/1 -> Vertical vel/1, Z/1  "Zdot"
  Z/1 -> Vertical disp/1  "Z"
  Susp Forces/1 -> Demux/1
  Demux/1 -> Sum of susp forces/1
  Demux/2 -> Sum of susp forces/2
  Demux/3 -> Sum of susp forces/3
  Demux/4 -> Sum of susp forces/4
  Sum of susp forces/1 -> Divide/1
  Divide/1 -> Sum5/2
  Gravity/1 -> Sum5/1
  Mass/1 -> Divide/2

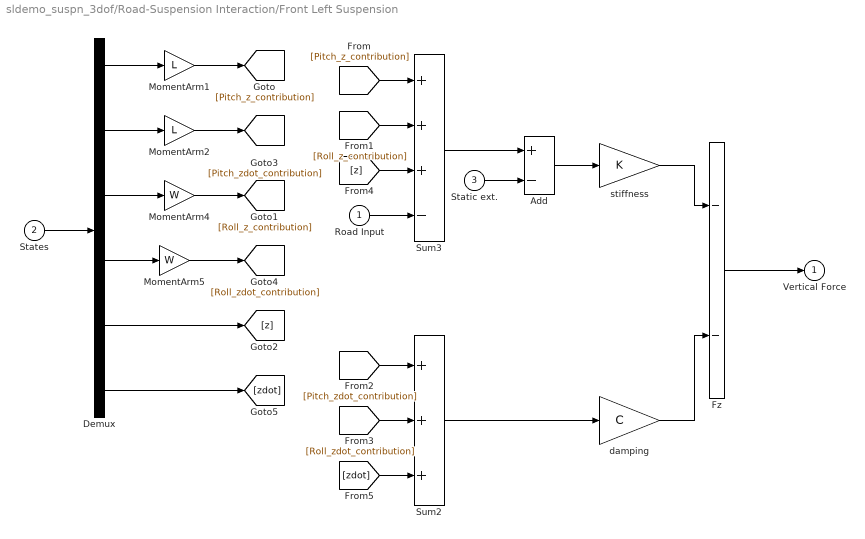
== system sldemo_suspn_3dof/Road-Suspension Interaction/Front Left Suspension ==
  Road Input : Inport
  States : Inport  Port=2
  Static ext. : Inport  Port=3
  Add : Sum  Inputs=+-
  Demux : Demux  Outputs=6
  Fz : Sum  Inputs=--  SaturateOnIntegerOverflow=on  InputSameDT=on  OutDataTypeStr=Inherit: Same as first input
  MomentArm1 : Gain  Gain=L  SaturateOnIntegerOverflow=on  OutDataTypeStr=Inherit: Same as input  ParamDataTypeStr=Inherit: Same as input
  MomentArm2 : Gain  Gain=L  SaturateOnIntegerOverflow=on  OutDataTypeStr=Inherit: Same as input  ParamDataTypeStr=Inherit: Same as input
  MomentArm4 : Gain  Gain=W  SaturateOnIntegerOverflow=on  OutDataTypeStr=Inherit: Same as input  ParamDataTypeStr=Inherit: Same as input
  MomentArm5 : Gain  Gain=W  SaturateOnIntegerOverflow=on  OutDataTypeStr=Inherit: Same as input  ParamDataTypeStr=Inherit: Same as input
  Sum2 : Sum  Inputs=+++  SaturateOnIntegerOverflow=on  InputSameDT=on  OutDataTypeStr=Inherit: Same as first input
  Sum3 : Sum  Inputs=+++-  SaturateOnIntegerOverflow=on  InputSameDT=on  OutDataTypeStr=Inherit: Same as first input
  damping : Gain  Gain=C  SaturateOnIntegerOverflow=on  OutDataTypeStr=Inherit: Same as input  ParamDataTypeStr=Inherit: Same as input
  stiffness : Gain  Gain=K  SaturateOnIntegerOverflow=on  OutDataTypeStr=Inherit: Same as input  ParamDataTypeStr=Inherit: Same as input
  Vertical Force : Outport
  wires:
  Sum2/1 -> damping/1
  States/1 -> Demux/1
  damping/1 -> Fz/2
  stiffness/1 -> Fz/1
  Demux/1 -> MomentArm1/1
  Demux/2 -> MomentArm2/1
  Fz/1 -> Vertical Force/1
  Demux/3 -> MomentArm4/1
  Demux/4 -> MomentArm5/1
  Sum3/1 -> Add/1
  Add/1 -> stiffness/1
  MomentArm1/1 -> [Pitch_z_contribution]
  MomentArm4/1 -> [Roll_z_contribution]
  Demux/5 -> [z]
  MomentArm2/1 -> [Pitch_zdot_contribution]
  MomentArm5/1 -> [Roll_zdot_contribution]
  Demux/6 -> [zdot]
  [Pitch_zdot_contribution] -> Sum2/1
  [Roll_zdot_contribution] -> Sum2/2
  [Pitch_z_contribution] -> Sum3/1
  [Roll_z_contribution] -> Sum3/2
  [z] -> Sum3/3
  [zdot] -> Sum2/3
  Road Input/1 -> Sum3/4
  Static ext./1 -> Add/2

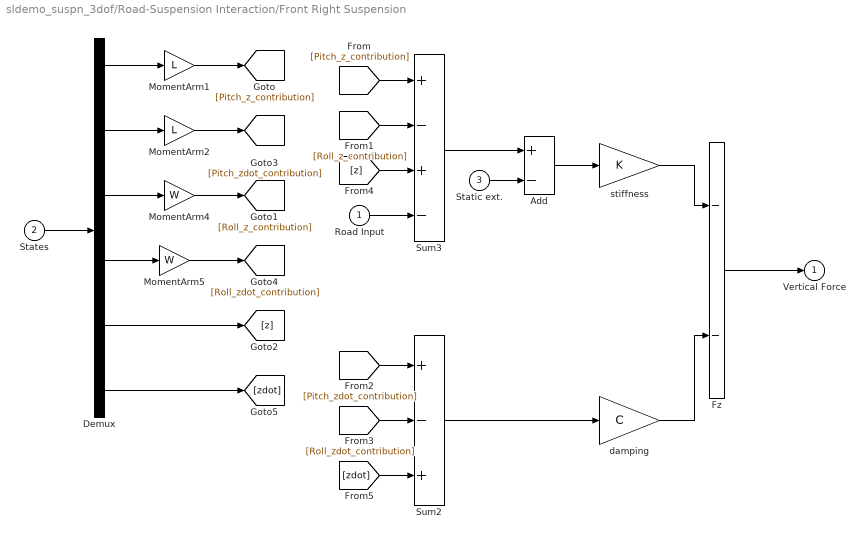
== system sldemo_suspn_3dof/Road-Suspension Interaction/Front Right Suspension ==
  Road Input : Inport
  States : Inport  Port=2
  Static ext. : Inport  Port=3
  Add : Sum  Inputs=+-
  Demux : Demux  Outputs=6
  Fz : Sum  Inputs=--  SaturateOnIntegerOverflow=on  InputSameDT=on  OutDataTypeStr=Inherit: Same as first input
  MomentArm1 : Gain  Gain=L  SaturateOnIntegerOverflow=on  OutDataTypeStr=Inherit: Same as input  ParamDataTypeStr=Inherit: Same as input
  MomentArm2 : Gain  Gain=L  SaturateOnIntegerOverflow=on  OutDataTypeStr=Inherit: Same as input  ParamDataTypeStr=Inherit: Same as input
  MomentArm4 : Gain  Gain=W  SaturateOnIntegerOverflow=on  OutDataTypeStr=Inherit: Same as input  ParamDataTypeStr=Inherit: Same as input
  MomentArm5 : Gain  Gain=W  SaturateOnIntegerOverflow=on  OutDataTypeStr=Inherit: Same as input  ParamDataTypeStr=Inherit: Same as input
  Sum2 : Sum  Inputs=+-+  SaturateOnIntegerOverflow=on  InputSameDT=on  OutDataTypeStr=Inherit: Same as first input
  Sum3 : Sum  Inputs=+-+-  SaturateOnIntegerOverflow=on  InputSameDT=on  OutDataTypeStr=Inherit: Same as first input
  damping : Gain  Gain=C  SaturateOnIntegerOverflow=on  OutDataTypeStr=Inherit: Same as input  ParamDataTypeStr=Inherit: Same as input
  stiffness : Gain  Gain=K  SaturateOnIntegerOverflow=on  OutDataTypeStr=Inherit: Same as input  ParamDataTypeStr=Inherit: Same as input
  Vertical Force : Outport
  wires:
  Sum2/1 -> damping/1
  States/1 -> Demux/1
  damping/1 -> Fz/2
  stiffness/1 -> Fz/1
  Demux/1 -> MomentArm1/1
  Demux/2 -> MomentArm2/1
  Fz/1 -> Vertical Force/1
  Demux/3 -> MomentArm4/1
  Demux/4 -> MomentArm5/1
  Sum3/1 -> Add/1
  Add/1 -> stiffness/1
  MomentArm1/1 -> [Pitch_z_contribution]
  MomentArm4/1 -> [Roll_z_contribution]
  Demux/5 -> [z]
  MomentArm2/1 -> [Pitch_zdot_contribution]
  MomentArm5/1 -> [Roll_zdot_contribution]
  Demux/6 -> [zdot]
  [Pitch_zdot_contribution] -> Sum2/1
  [Roll_zdot_contribution] -> Sum2/2
  [Pitch_z_contribution] -> Sum3/1
  [Roll_z_contribution] -> Sum3/2
  [z] -> Sum3/3
  [zdot] -> Sum2/3
  Road Input/1 -> Sum3/4
  Static ext./1 -> Add/2

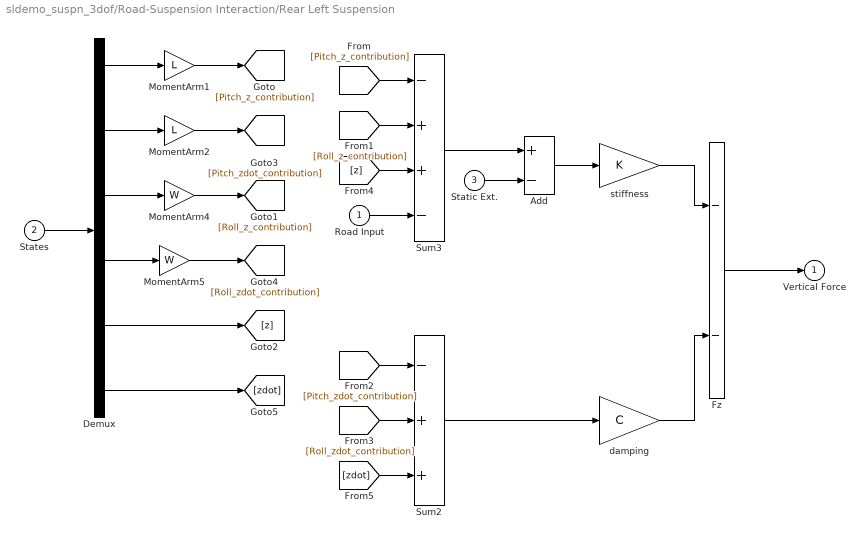
== system sldemo_suspn_3dof/Road-Suspension Interaction/Rear Left Suspension ==
  Road Input : Inport
  States : Inport  Port=2
  Static Ext. : Inport  Port=3
  Add : Sum  Inputs=+-
  Demux : Demux  Outputs=6
  Fz : Sum  Inputs=--  SaturateOnIntegerOverflow=on  InputSameDT=on  OutDataTypeStr=Inherit: Same as first input
  MomentArm1 : Gain  Gain=L  SaturateOnIntegerOverflow=on  OutDataTypeStr=Inherit: Same as input  ParamDataTypeStr=Inherit: Same as input
  MomentArm2 : Gain  Gain=L  SaturateOnIntegerOverflow=on  OutDataTypeStr=Inherit: Same as input  ParamDataTypeStr=Inherit: Same as input
  MomentArm4 : Gain  Gain=W  SaturateOnIntegerOverflow=on  OutDataTypeStr=Inherit: Same as input  ParamDataTypeStr=Inherit: Same as input
  MomentArm5 : Gain  Gain=W  SaturateOnIntegerOverflow=on  OutDataTypeStr=Inherit: Same as input  ParamDataTypeStr=Inherit: Same as input
  Sum2 : Sum  Inputs=-++  SaturateOnIntegerOverflow=on  InputSameDT=on  OutDataTypeStr=Inherit: Same as first input
  Sum3 : Sum  Inputs=-++-  SaturateOnIntegerOverflow=on  InputSameDT=on  OutDataTypeStr=Inherit: Same as first input
  damping : Gain  Gain=C  SaturateOnIntegerOverflow=on  OutDataTypeStr=Inherit: Same as input  ParamDataTypeStr=Inherit: Same as input
  stiffness : Gain  Gain=K  SaturateOnIntegerOverflow=on  OutDataTypeStr=Inherit: Same as input  ParamDataTypeStr=Inherit: Same as input
  Vertical Force : Outport
  wires:
  Road Input/1 -> Sum3/4
  [zdot] -> Sum2/3
  [z] -> Sum3/3
  [Roll_z_contribution] -> Sum3/2
  [Pitch_z_contribution] -> Sum3/1
  [Roll_zdot_contribution] -> Sum2/2
  [Pitch_zdot_contribution] -> Sum2/1
  Demux/6 -> [zdot]
  MomentArm5/1 -> [Roll_zdot_contribution]
  MomentArm2/1 -> [Pitch_zdot_contribution]
  Demux/5 -> [z]
  MomentArm4/1 -> [Roll_z_contribution]
  MomentArm1/1 -> [Pitch_z_contribution]
  Add/1 -> stiffness/1
  Sum3/1 -> Add/1
  Demux/4 -> MomentArm5/1
  Demux/3 -> MomentArm4/1
  Fz/1 -> Vertical Force/1
  Demux/2 -> MomentArm2/1
  Demux/1 -> MomentArm1/1
  stiffness/1 -> Fz/1
  damping/1 -> Fz/2
  States/1 -> Demux/1
  Sum2/1 -> damping/1
  Static Ext./1 -> Add/2

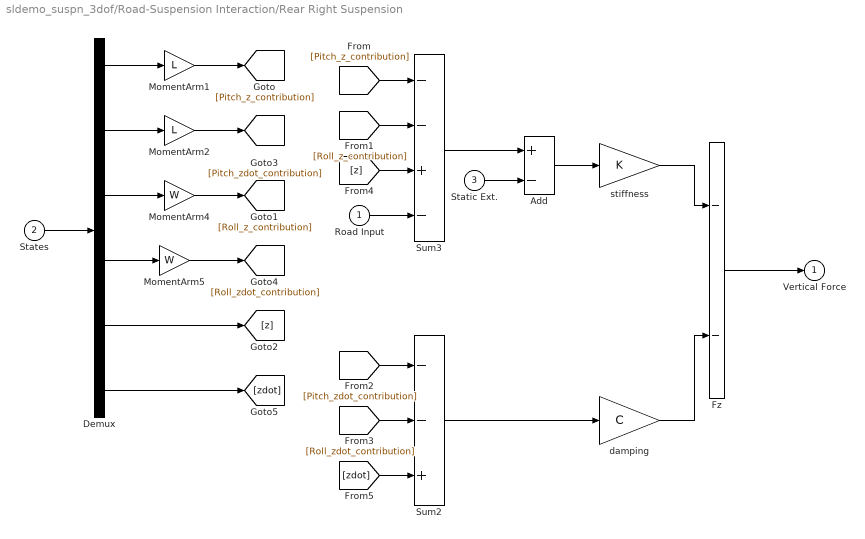
== system sldemo_suspn_3dof/Road-Suspension Interaction/Rear Right Suspension ==
  Road Input : Inport
  States : Inport  Port=2
  Static Ext. : Inport  Port=3
  Add : Sum  Inputs=+-
  Demux : Demux  Outputs=6
  Fz : Sum  Inputs=--  SaturateOnIntegerOverflow=on  InputSameDT=on  OutDataTypeStr=Inherit: Same as first input
  MomentArm1 : Gain  Gain=L  SaturateOnIntegerOverflow=on  OutDataTypeStr=Inherit: Same as input  ParamDataTypeStr=Inherit: Same as input
  MomentArm2 : Gain  Gain=L  SaturateOnIntegerOverflow=on  OutDataTypeStr=Inherit: Same as input  ParamDataTypeStr=Inherit: Same as input
  MomentArm4 : Gain  Gain=W  SaturateOnIntegerOverflow=on  OutDataTypeStr=Inherit: Same as input  ParamDataTypeStr=Inherit: Same as input
  MomentArm5 : Gain  Gain=W  SaturateOnIntegerOverflow=on  OutDataTypeStr=Inherit: Same as input  ParamDataTypeStr=Inherit: Same as input
  Sum2 : Sum  Inputs=--+  SaturateOnIntegerOverflow=on  InputSameDT=on  OutDataTypeStr=Inherit: Same as first input
  Sum3 : Sum  Inputs=--+-  SaturateOnIntegerOverflow=on  InputSameDT=on  OutDataTypeStr=Inherit: Same as first input
  damping : Gain  Gain=C  SaturateOnIntegerOverflow=on  OutDataTypeStr=Inherit: Same as input  ParamDataTypeStr=Inherit: Same as input
  stiffness : Gain  Gain=K  SaturateOnIntegerOverflow=on  OutDataTypeStr=Inherit: Same as input  ParamDataTypeStr=Inherit: Same as input
  Vertical Force : Outport
  wires:
  Road Input/1 -> Sum3/4
  [zdot] -> Sum2/3
  [z] -> Sum3/3
  [Roll_z_contribution] -> Sum3/2
  [Pitch_z_contribution] -> Sum3/1
  [Roll_zdot_contribution] -> Sum2/2
  [Pitch_zdot_contribution] -> Sum2/1
  Demux/6 -> [zdot]
  MomentArm5/1 -> [Roll_zdot_contribution]
  MomentArm2/1 -> [Pitch_zdot_contribution]
  Demux/5 -> [z]
  MomentArm4/1 -> [Roll_z_contribution]
  MomentArm1/1 -> [Pitch_z_contribution]
  Add/1 -> stiffness/1
  Sum3/1 -> Add/1
  Demux/4 -> MomentArm5/1
  Demux/3 -> MomentArm4/1
  Fz/1 -> Vertical Force/1
  Demux/2 -> MomentArm2/1
  Demux/1 -> MomentArm1/1
  stiffness/1 -> Fz/1
  damping/1 -> Fz/2
  States/1 -> Demux/1
  Sum2/1 -> damping/1
  Static Ext./1 -> Add/2
